simulink model "Model_DCmotor_FinalExamED"  (R2020b)
settings: Solver=FixedStepAuto  StartTime=0.0  StopTime=100.0  FixedStep=SampleTime  MaxStep=1e-5  RelTol=1e-3
values from neighbouring files (symbols this model uses):
  Capacitance = 10e-3    (= 0.01)    [Parameters.m]
  CarrierFrequency = 1e-3    (= 0.001)    [Parameters.m]
  ConverterMAXoutCurrent = 1.4    [Parameters.m]
  Current_KI = 0.00025    [Parameters.m]
  Current_KP = 26331    [Parameters.m]
  Inductance = 9.31e-3    (= 0.00931)    [Parameters.m]
  LoadTorqueSlope = 1.6e-3    (= 0.0016)    [Parameters.m]
  Resistance = 37.10    (= 37.1)    [Parameters.m]
  Speed_KI = 0.415    [Parameters.m]
  Speed_KP = 1.0    (= 1)    [Parameters.m]
  SpeedCONSTANT = 29.8*(2*pi/60)    (= 3.12064870257)    [Parameters.m]
  SupplyInternalInductance = 0.4e-3    (= 0.0004)    [Parameters.m]
  SupplyInternalResistance = 0.4    [Parameters.m]
  SupplyVoltage = 80    [Parameters.m]
  TorqueCONSTANT = 0.321    [Parameters.m]
  TotalInertia = (RotorInertia+LoadInertia)    (= 2.8e-05)    [Parameters.m]
undefined symbols (not defined in the file or in its folder): CapacitanceResistance
libraries: powerlib x27, simulink x5
settings Model: Creator=Baraghini Nicholas  LastModifiedBy=Baraghini Nicholas
settings SolverCC: ZeroCrossAlgorithm=Adaptive
settings DataIOCC: Refine=1.5
settings DebuggingCC: MaskedZcDiagnostic=none  IgnoredZcDiagnostic=none

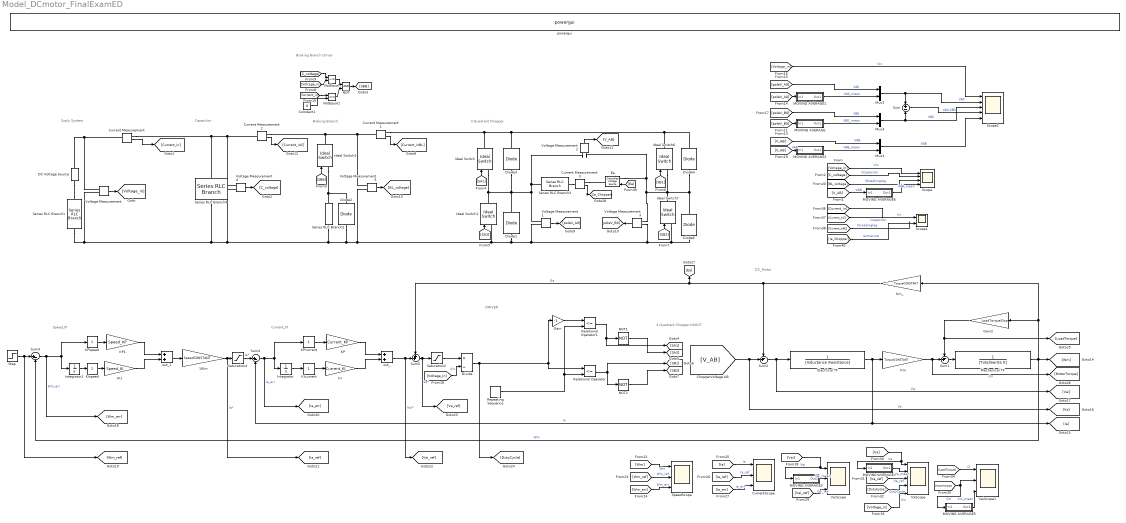
== system Model_DCmotor_FinalExamED ==
  note: Braking Branch Driver
  note: 4 Quadrant Chopper IN/OUT
  note: 4 Quadrant Chopper
  note: Suply System
  note: Capacitor
  note: Braking Branch
  note: DRIVER
  note: Speed_PI
  note: Current_PI
  note: DC_Motor
  1/Km : Gain  Gain=SpeedCONSTANT
  Constant1 : Constant  Value=0
  Current Measurement{,1..3} (4 alike) : powerlib/Measurements/Current Measurement  PhasorSimulation=off  OutputType=Complex  PSBequivalent=0
  CurrentScope : Scope  NumInputPorts=3
  DC Voltage Source : powerlib/Electrical Sources/DC Voltage Source  Amplitude=SupplyVoltage  Measurements=None
  Diode{1..5} (5 alike) : powerlib/Power Electronics/Diode  Ron=DiodeResistance  Lon=0  Vf=DiodeVfm  IC=0  UseSnubber=0  Rs=DiodeResistance  Cs=inf  Measurements=off
  Divide : Product  Inputs=*/
  Ea : powerlib/Electrical Sources/Controlled Voltage Source  Initialize=on  Source_Type=DC  Amplitude=0  Phase=0  Frequency=0  Measurements=None
  Electrical TF : TransferFcn  Denominator=[Inductance Resistance]
  Gain : Gain  Gain=-1
  Gain2 : Gain  Gain=LoadTorqueSlope
  Ideal Switch{,1..2,6..7} (5 alike) : powerlib/Power Electronics/Ideal Switch  Ron=MosfetResistance  Lon=0  IC=0  Rs=DiodeResistance  Cs=inf  Measurements=off
  Integrator : Integrator
  Integrator1 : Integrator
  KI : Gain  Gain=Current_KI
  KI1 : Gain  Gain=Speed_KI
  KIcurrent : simulink/Math Operations/Slider Gain  gain=1  low=0  high=1e9
  KIspeed : simulink/Math Operations/Slider Gain  gain=1  low=0  high=1e9
  KP : Gain  Gain=Current_KP
  KP1 : Gain  Gain=Speed_KP
  KPcurrent : simulink/Math Operations/Slider Gain  gain=1  low=0  high=1e9
  KPspeed : simulink/Math Operations/Slider Gain  gain=1  low=0  high=1e9
  Km : Gain  Gain=TorqueCONSTANT
  Km_ : Gain  Gain=TorqueCONSTANT
  MOVING AVERAGE : Subsystem
  MOVING AVERAGE1 : Subsystem
  MOVING AVERAGE2 : Subsystem
  MOVING AVERAGE3 : Subsystem
  MOVING AVERAGE4 : Subsystem
  MOVING AVERAGE5 : Subsystem
  MOVING AVERAGE6 : Subsystem
  Mechanical TF : TransferFcn  Denominator=[TotalInertia 0]
  Mux2 : Mux  Inputs=2
  Mux3 : Mux  Inputs=2
  Mux4 : Mux  Inputs=2
  NOT : Logic  IconShape=distinctive  AllPortsSameDT=off  OutDataTypeStr=boolean
  NOT1 : Logic  Operator=NOT  IconShape=distinctive  AllPortsSameDT=off  OutDataTypeStr=boolean
  NOT2 : Logic  Operator=NOT  IconShape=distinctive  AllPortsSameDT=off  OutDataTypeStr=boolean
  NotEqual : RelationalOperator  Operator=~=  OutDataTypeStr=boolean  RndMeth=Simplest
  NotEqual1 : RelationalOperator  Operator=<=  OutDataTypeStr=boolean  RndMeth=Simplest
  Relational Operator : RelationalOperator  Operator=<=  OutDataTypeStr=boolean  RndMeth=Simplest
  Relational Operator1 : RelationalOperator  Operator=<=  OutDataTypeStr=boolean  RndMeth=Simplest
  Repeating Sequence : simulink/Sources/Repeating Sequence  rep_seq_t=[0 (CarrierFrequency)/2 CarrierFrequency]  rep_seq_y=[-1 1 -1]
  Saturation2 : Saturate  UpperLimit=79.94  LowerLimit=-79.94
  Saturation4 : Saturate  UpperLimit=ConverterMAXoutCurrent  LowerLimit=-ConverterMAXoutCurrent
  Scope : Scope  NumInputPorts=4
  Scope1 : Scope  NumInputPorts=2
  Scope2 : Scope  NumInputPorts=5
  Series RLC Branch1 : powerlib/Elements/Series RLC Branch  LConnTagsString=__new0  RConnTagsString=__new0  BranchType=RL  Resistance=SupplyInternalResistance  Inductance=SupplyInternalInductance  SetiL0=off  InitialCurrent=0  Capacitance=1  Setx0=off  InitialVoltage=0  Measurements=None
  Series RLC Branch2 : powerlib/Elements/Series RLC Branch  LConnTagsString=__new0  RConnTagsString=__new0  BranchType=R  Resistance=10  Inductance=10e-3  SetiL0=off  InitialCurrent=0  Capacitance=1  Setx0=off  InitialVoltage=0  Measurements=None
  Series RLC Branch3 : powerlib/Elements/Series RLC Branch  LConnTagsString=__new0  RConnTagsString=__new0  BranchType=RL  Resistance=Resistance  Inductance=Inductance  SetiL0=off  InitialCurrent=0  Capacitance=1  Setx0=off  InitialVoltage=0  Measurements=None
  Series RLC Branch4 : powerlib/Elements/Series RLC Branch  LConnTagsString=__new0  RConnTagsString=__new0  BranchType=C  Resistance=CapacitanceResistance  Inductance=10e-3  SetiL0=off  InitialCurrent=0  Capacitance=Capacitance  Setx0=on  InitialVoltage=0  Measurements=None
  SpeedScope : Scope  NumInputPorts=3
  Step : Step  Time=0  After=81  SampleTime=0
  Sum : Sum  Inputs=+-
  Sum1 : Sum  Inputs=-+|
  Sum2 : Sum  Inputs=-+|
  Sum3 : Sum  Inputs=|+-
  Sum4 : Sum  Inputs=|+-
  Sum5 : Sum  Inputs=++|
  VaScope : Scope  NumInputPorts=5
  VaiScope : Scope  NumInputPorts=3
  VaiScope1 : Scope  NumInputPorts=3
  Voltage Measurement{,1..5} (6 alike) : powerlib/Measurements/Voltage Measurement  PhasorSimulation=off  OutputType=Complex  PSBequivalent=0
  out_ : Sum
  out_1 : Sum
  powergui : powerlib/powergui  Priority=1  SimulationMode=Continuous  SampleTime=50e-6  frequency=60  Iterations=50  frequencyindice=0  Pbase=100e6  ErrMax=1e-4  UnitsV=kV  UnitsW=MW  buscounter=0  FunctionMessages=off  echomessages=off  EnableUseOfTLC=off  CurrentSourceSwitches=off  DisableSnubberDevices=off  DisableRonSwitches=off  DisableVfSwitches=off  DisplayEquations=off  AutomaticDiscreteSolvers=off  SolverType=Tustin/Backward Euler (TBE)  Interpol=off  ExternalGateDelay=off  methode=off  Ts=100  x0status=blocks  SPID=on  SwTol=0  HookPort=off  NonlinearTolerance=1e-4  nMaxIteration=100  ContinueOnMaxIteration=off  RestoreLinks=warning  ResistiveCurrentMeasurement=off  Frange=[0:2:500]  Ylog=off  Xlog=on  ShowGrid=off  save=off  variable=ZData  structure=0  ZoomFFT=off  StartTime=0.0  cycles=1  DisplayStyle=1  fundamental=60  FreqAxis=off  MaxFrequency=1000  frequencyindicesteady=1  RmsSteady=1  display=off
  wires:
  [SB2] -> Ideal Switch7/1
  [SA2] -> Ideal Switch1/1
  NOT2/1 -> [SB2]
  NOT1/1 -> [SA2]
  [SB1] -> Ideal Switch6/1
  Relational Operator/1 -> [SB1], NOT2/1
  [Voltage_in] -> Scope/1  "Vin"
  Voltage Measurement/1 -> [Voltage_in]
  Relational Operator1/1 -> [SA1], NOT1/1
  Current Measurement/1 -> [Current_in]
  [SA1] -> Ideal Switch/1
  [Voltage_in] -> NotEqual/2
  NotEqual/1 -> NOT/1
  [C_voltage] -> NotEqual/1
  NotEqual1/1 -> NOT/2
  [Current_in] -> NotEqual1/1
  Constant1/1 -> NotEqual1/2
  Voltage Measurement4/1 -> [C_voltage]
  [C_voltage] -> Scope/2  "Vcapacitor"
  NOT/1 -> [SBB]
  [SBB] -> Ideal Switch2/1
  Current Measurement1/1 -> [Current_inBL]
  Voltage Measurement1/1 -> [poleV_A0]
  Voltage Measurement3/1 -> [poleV_B0]
  [poleV_A0] -> Mux2/1  "VA0"
  [poleV_B0] -> Mux3/1  "VB0"
  [Voltage_in] -> Scope2/1  "Vin"
  Mux2/1 -> Sum/1, Scope2/2  "VA0"
  Mux3/1 -> Sum/2, Scope2/3  "VB0"
  MOVING AVERAGE/1(Out1) -> Mux3/2  "VB0_mean"
  [poleV_B0] -> MOVING AVERAGE/1(In1)
  [poleV_A0] -> MOVING AVERAGE1/1(In1)
  MOVING AVERAGE1/1(Out1) -> Mux2/2  "VA0_mean"
  Sum/1 -> Scope2/4  "VA0-VB0"
  Sum2/1 -> [Vai], Electrical TF/1  "Vai"
  [V_AB] -> [Va], Sum2/2  "Va"
  Electrical TF/1 -> Sum4/2, [Ia], Km/1  "Ia"
  Sum1/1 -> Mechanical TF/1
  Mechanical TF/1 -> [Wm], Km_/1, Gain2/1, Sum3/2  "Wm"
  Km_/1 -> Sum5/1, [Ea], Sum2/1  "Ea"
  Gain2/1 -> Sum1/1, [LoadTorque]
  Voltage Measurement2/1 -> [V_AB]
  Sum3/1 -> [Wm_err], KPspeed/1, Integrator1/1  "Wm_err"
  Sum4/1 -> [Ia_err], KPcurrent/1, Integrator/1  "Ia_err"
  out_1/1 -> 1/Km/1
  1/Km/1 -> [Ia_ref], Saturation4/1  "Ia*"
  out_/1 -> [Vai_ref], Sum5/2  "Vai*"
  [Voltage_in] -> Divide/2  "Vin"
  Step/1 -> [Wm_ref], Sum3/1
  Sum5/1 -> Saturation2/1, [Va_ref]  "Va*"
  KP/1 -> out_/1
  KI/1 -> out_/2
  Integrator/1 -> KIcurrent/1
  Integrator1/1 -> KIspeed/1
  KI1/1 -> out_1/2
  KP1/1 -> out_1/1
  Saturation2/1 -> Divide/1
  Km/1 -> [MotorTorque], Sum1/2  "Cm"
  Saturation4/1 -> Sum4/1  "Ia*"
  KPcurrent/1 -> KP/1
  KIcurrent/1 -> KI/1
  KPspeed/1 -> KP1/1
  KIspeed/1 -> KI1/1
  Divide/1 -> [DutyCycle], Relational Operator/1, Gain/1
  Gain/1 -> Relational Operator1/1
  Repeating Sequence/1 -> Relational Operator1/2, Relational Operator/2
  MOVING AVERAGE2/1(Out1) -> Mux4/2  "VAB_mean"
  [V_AB] -> Mux4/1  "VAB"
  [V_AB] -> MOVING AVERAGE2/1(In1)  "VAB"
  Mux4/1 -> Scope2/5  "VAB"
  Current Measurement2/1 -> [Current_inC]
  Voltage Measurement5/1 -> [BL_voltage]
  [BL_voltage] -> Scope/3  "Vbreakingleg"
  [Wm] -> SpeedScope/1  "Wm"
  [Wm_ref] -> SpeedScope/2  "Wm_ref"
  [Wm_err] -> SpeedScope/3  "Wm_err"
  [Ia_err] -> CurrentScope/3  "Ia_err"
  [Ia_ref] -> CurrentScope/2  "Ia_ref"
  [Ia] -> CurrentScope/1  "Ia"
  [Vai_ref] -> VaiScope/3  "Vai_ref"
  [Va_ref] -> VaScope/3  "Va_ref"
  [Va] -> MOVING AVERAGE4/1(In1), VaScope/1  "Va"
  [DutyCycle] -> VaScope/4  "DutyCycle"
  [Voltage_in] -> VaScope/5  "Vin"
  [MotorTorque] -> MOVING AVERAGE5/1(In1), VaiScope1/2  "Cm"
  [LoadTorque] -> VaiScope1/1  "Cl"
  MOVING AVERAGE3/1(Out1) -> VaiScope/2  "Vai_mean"
  [Vai] -> MOVING AVERAGE3/1(In1), VaiScope/1  "Vai"
  MOVING AVERAGE4/1(Out1) -> VaScope/2  "Va_mean"
  MOVING AVERAGE5/1(Out1) -> VaiScope1/3  "Cm_mean"
  [Current_inBL] -> ?  "Ibreakingleg"
  [Current_inC] -> ?  "Icapacitor"
  [Current_in] -> Scope1/1  "Iin"
  [Ea] -> Ea/1
  Current Measurement3/1 -> [Ia_Chopper]
  [Ia_Chopper] -> Scope1/2  "Iarmature"
  [V_AB] -> MOVING AVERAGE6/1(In1)  "VAB"
  MOVING AVERAGE6/1(Out1) -> Scope/4  "VAB_mean"
  connections:
  Ideal Switch6/RConn1 -- Diode4/RConn1 -- Diode3/RConn1 -- Current Measurement1/RConn1 -- Ideal Switch/RConn1
  Ideal Switch6/LConn1 -- Ea/LConn1 -- Voltage Measurement2/LConn2 -- Voltage Measurement3/LConn1 -- Diode4/LConn1 -- Diode5/RConn1 -- Ideal Switch7/RConn1
  Ideal Switch7/LConn1 -- Voltage Measurement3/LConn2 -- Voltage Measurement1/LConn2 -- Diode1/LConn1 -- Voltage Measurement5/LConn2 -- Voltage Measurement4/LConn2 -- Voltage Measurement/LConn2 -- Series RLC Branch1/RConn1 -- Series RLC Branch4/RConn1 -- Series RLC Branch2/RConn1 -- Diode2/LConn1 -- Ideal Switch1/LConn1 -- Diode5/LConn1
  DC Voltage Source/RConn1 -- Current Measurement/LConn1 -- Voltage Measurement/LConn1
  Ideal Switch/LConn1 -- Diode1/RConn1 -- Diode3/LConn1 -- Voltage Measurement2/LConn1 -- Series RLC Branch3/LConn1 -- Voltage Measurement1/LConn1 -- Ideal Switch1/RConn1
  Ideal Switch2/LConn1 -- Diode2/RConn1 -- Series RLC Branch2/LConn1
  DC Voltage Source/LConn1 -- Series RLC Branch1/LConn1
  Current Measurement1/LConn1 -- Voltage Measurement5/LConn1 -- Current Measurement2/RConn1 -- Ideal Switch2/RConn1
  Voltage Measurement4/LConn1 -- Current Measurement2/LConn1 -- Current Measurement/RConn1 -- Series RLC Branch4/LConn1
  Series RLC Branch3/RConn1 -- Current Measurement3/LConn1
  Current Measurement3/RConn1 -- Ea/RConn1

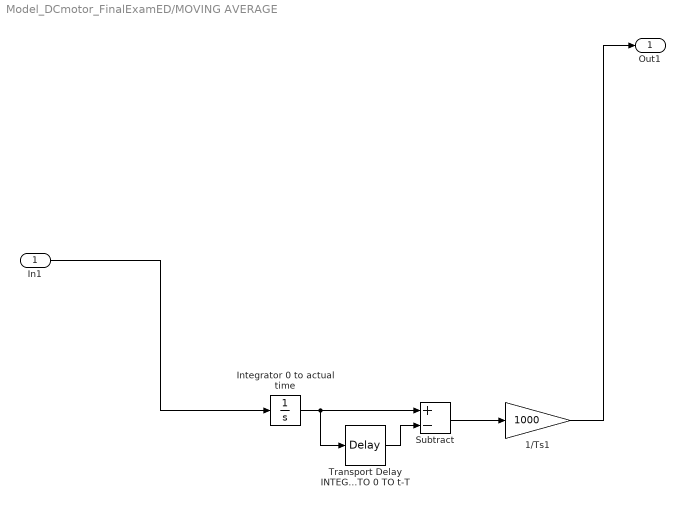
== system Model_DCmotor_FinalExamED/MOVING AVERAGE ==
  In1 : Inport
  1/Ts1 : Gain  Gain=1000
  "Integrator 0 to actual time " : Integrator
  Subtract : Sum  Inputs=+-
  Transport Delay INTEGRAL O TO 0 TO t-T : TransportDelay  DelayTime=1/1000
  Out1 : Outport  VectorParamsAs1DForOutWhenUnconnected=off
  wires:
  In1/1 -> "Integrator 0 to actual time "/1
  1/Ts1/1 -> Out1/1
  "Integrator 0 to actual time "/1 -> Transport Delay INTEGRAL O TO 0 TO t-T/1, Subtract/1
  Transport Delay INTEGRAL O TO 0 TO t-T/1 -> Subtract/2
  Subtract/1 -> 1/Ts1/1

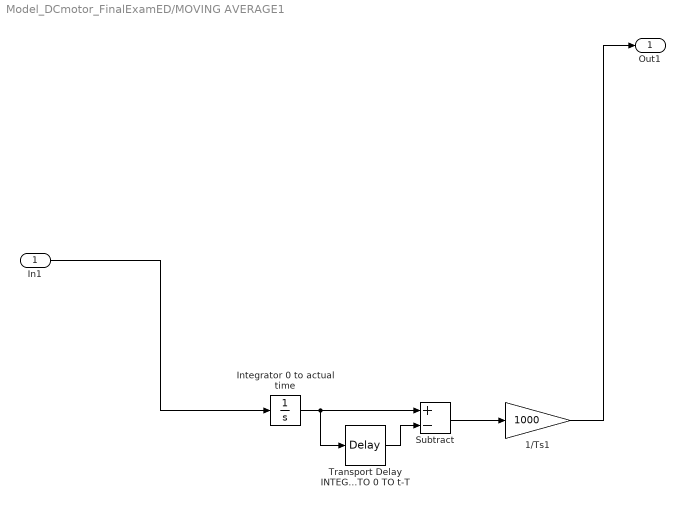
== system Model_DCmotor_FinalExamED/MOVING AVERAGE1 ==
  In1 : Inport
  1/Ts1 : Gain  Gain=1000
  "Integrator 0 to actual time " : Integrator
  Subtract : Sum  Inputs=+-
  Transport Delay INTEGRAL O TO 0 TO t-T : TransportDelay  DelayTime=1/1000
  Out1 : Outport  VectorParamsAs1DForOutWhenUnconnected=off
  wires:
  Subtract/1 -> 1/Ts1/1
  Transport Delay INTEGRAL O TO 0 TO t-T/1 -> Subtract/2
  "Integrator 0 to actual time "/1 -> Subtract/1, Transport Delay INTEGRAL O TO 0 TO t-T/1
  1/Ts1/1 -> Out1/1
  In1/1 -> "Integrator 0 to actual time "/1

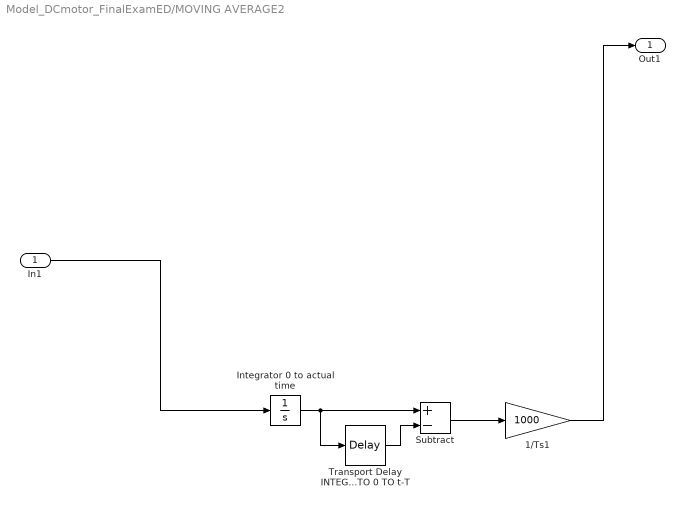
== system Model_DCmotor_FinalExamED/MOVING AVERAGE2 ==
  In1 : Inport
  1/Ts1 : Gain  Gain=1000
  "Integrator 0 to actual time " : Integrator
  Subtract : Sum  Inputs=+-
  Transport Delay INTEGRAL O TO 0 TO t-T : TransportDelay  DelayTime=1/1000
  Out1 : Outport  VectorParamsAs1DForOutWhenUnconnected=off
  wires:
  Subtract/1 -> 1/Ts1/1
  Transport Delay INTEGRAL O TO 0 TO t-T/1 -> Subtract/2
  "Integrator 0 to actual time "/1 -> Subtract/1, Transport Delay INTEGRAL O TO 0 TO t-T/1
  1/Ts1/1 -> Out1/1
  In1/1 -> "Integrator 0 to actual time "/1

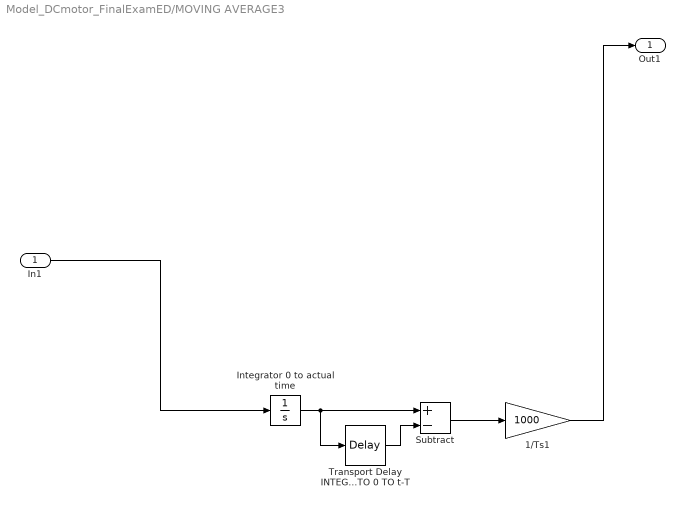
== system Model_DCmotor_FinalExamED/MOVING AVERAGE3 ==
  In1 : Inport
  1/Ts1 : Gain  Gain=1000
  "Integrator 0 to actual time " : Integrator
  Subtract : Sum  Inputs=+-
  Transport Delay INTEGRAL O TO 0 TO t-T : TransportDelay  DelayTime=1/1000
  Out1 : Outport  VectorParamsAs1DForOutWhenUnconnected=off
  wires:
  In1/1 -> "Integrator 0 to actual time "/1
  1/Ts1/1 -> Out1/1
  "Integrator 0 to actual time "/1 -> Transport Delay INTEGRAL O TO 0 TO t-T/1, Subtract/1
  Transport Delay INTEGRAL O TO 0 TO t-T/1 -> Subtract/2
  Subtract/1 -> 1/Ts1/1

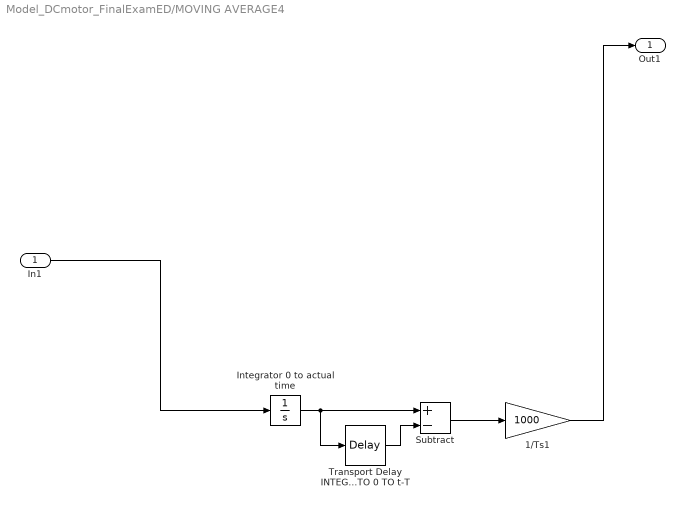
== system Model_DCmotor_FinalExamED/MOVING AVERAGE4 ==
  In1 : Inport
  1/Ts1 : Gain  Gain=1000
  "Integrator 0 to actual time " : Integrator
  Subtract : Sum  Inputs=+-
  Transport Delay INTEGRAL O TO 0 TO t-T : TransportDelay  DelayTime=1/1000
  Out1 : Outport  VectorParamsAs1DForOutWhenUnconnected=off
  wires:
  Subtract/1 -> 1/Ts1/1
  Transport Delay INTEGRAL O TO 0 TO t-T/1 -> Subtract/2
  "Integrator 0 to actual time "/1 -> Subtract/1, Transport Delay INTEGRAL O TO 0 TO t-T/1
  1/Ts1/1 -> Out1/1
  In1/1 -> "Integrator 0 to actual time "/1

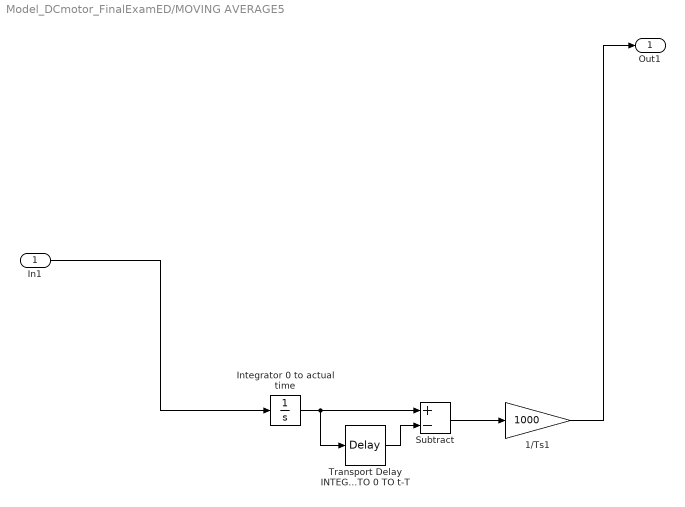
== system Model_DCmotor_FinalExamED/MOVING AVERAGE5 ==
  In1 : Inport
  1/Ts1 : Gain  Gain=1000
  "Integrator 0 to actual time " : Integrator
  Subtract : Sum  Inputs=+-
  Transport Delay INTEGRAL O TO 0 TO t-T : TransportDelay  DelayTime=1/1000
  Out1 : Outport  VectorParamsAs1DForOutWhenUnconnected=off
  wires:
  In1/1 -> "Integrator 0 to actual time "/1
  1/Ts1/1 -> Out1/1
  "Integrator 0 to actual time "/1 -> Transport Delay INTEGRAL O TO 0 TO t-T/1, Subtract/1
  Transport Delay INTEGRAL O TO 0 TO t-T/1 -> Subtract/2
  Subtract/1 -> 1/Ts1/1

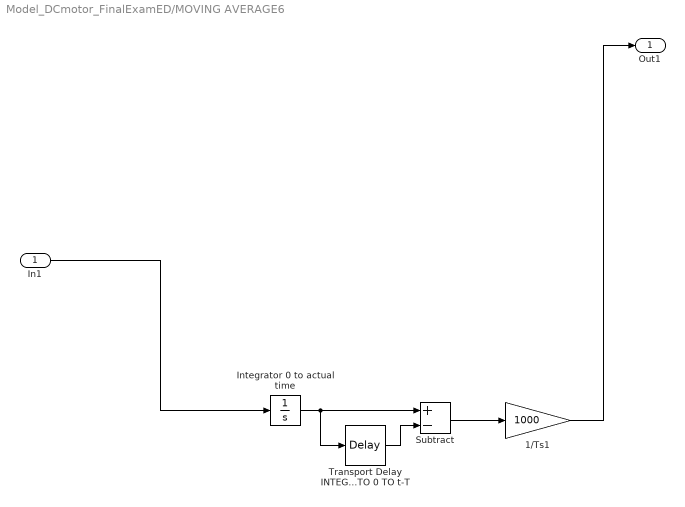
== system Model_DCmotor_FinalExamED/MOVING AVERAGE6 ==
  In1 : Inport
  1/Ts1 : Gain  Gain=1000
  "Integrator 0 to actual time " : Integrator
  Subtract : Sum  Inputs=+-
  Transport Delay INTEGRAL O TO 0 TO t-T : TransportDelay  DelayTime=1/1000
  Out1 : Outport  VectorParamsAs1DForOutWhenUnconnected=off
  wires:
  In1/1 -> "Integrator 0 to actual time "/1
  1/Ts1/1 -> Out1/1
  "Integrator 0 to actual time "/1 -> Transport Delay INTEGRAL O TO 0 TO t-T/1, Subtract/1
  Transport Delay INTEGRAL O TO 0 TO t-T/1 -> Subtract/2
  Subtract/1 -> 1/Ts1/1
